simulink model "PickLead_Test"  (Simulink 7.8)
settings: Solver=ode45  StartTime=0.0  StopTime=50  RelTol=1e-3
libraries: simulink x1
settings Model: Creator=jmapatel  LastModifiedBy=cjzhang
settings OptimizationCC: InitFltsAndDblsToZero=on
settings DebuggingCC: SaveWithParameterizedLinksMsg=none  FcnCallInpInsideContextMsg=Use local settings  StrictBusMsg=Warning
settings GRTTargetCC: TargetFcnLib=ansi_tfl_tmw.mat

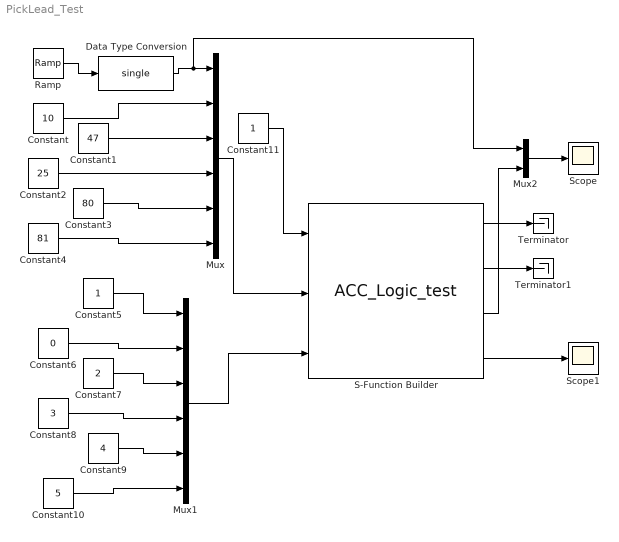
== system PickLead_Test ==
  Constant : Constant  Value=10  OutDataTypeStr=single
  Constant1 : Constant  Value=47  OutDataTypeStr=single
  Constant10 : Constant  Value=5  OutDataTypeStr=single
  Constant11 : Constant  OutDataTypeStr=boolean
  Constant2 : Constant  Value=25  OutDataTypeStr=single
  Constant3 : Constant  Value=80  OutDataTypeStr=single
  Constant4 : Constant  Value=81  OutDataTypeStr=single
  Constant5 : Constant  OutDataTypeStr=single
  Constant6 : Constant  Value=0  OutDataTypeStr=single
  Constant7 : Constant  Value=2  OutDataTypeStr=single
  Constant8 : Constant  Value=3  OutDataTypeStr=single
  Constant9 : Constant  Value=4  OutDataTypeStr=single
  Data Type Conversion : DataTypeConversion  OutDataTypeStr=single
  Mux : Mux  Inputs=6
  Mux1 : Mux  Inputs=6
  Mux2 : Mux  Inputs=2
  Ramp : simulink/Sources/Ramp  slope=2  start=0  X0=0
  S-Function Builder : S-Function  InitFcn=try, set_param(gcb,'FunctionName','ACC_Logic_test'), end  FunctionName=ACC_Logic_test  Parameters=1  SFunctionModules=ACC_Logic_test_wrapper  WizardData=DataTag0  EnableBusSupport=off
      mask init:
      | val = [[.9  0.75 0.75 1 1 .9 .9 1]',[1 1 0.75 0.75 .9 .9 1 .9]'];try , sys = get_param(gcb,'SfunBuilderFcnName');if isempty(sys), sys = get_param(gcb,'FunctionName'); end,catch, sys = get_param(gcb,'FunctionName'); end
      settings: CopyFcn=set_param(gcbh,'LinkStatus','none')  PreSaveFcn=try, set_param(gcb,'FunctionName','ACC_Logic_test'), end  OpenFcn=sfunctionwizard(gcbh)
      mask Display: plot(val(:,1),val(:,2)),disp(sys), port_label('input',1,'en_man'), port_label('input',2,'s'), port_label('input',3,'u'), port_label('output',1,'en_vel'), port_label('output',2,'en_pos'), port_label('output',3,'lead_s'), port_label('output',4,'lead_us')
  Scope : Scope
  Scope1 : Scope
  Terminator : Terminator
  Terminator1 : Terminator
  wires:
  Mux2/1 -> Scope/1
  Constant/1 -> Mux/2
  Constant1/1 -> Mux/3
  Constant2/1 -> Mux/4
  Constant3/1 -> Mux/5
  Constant4/1 -> Mux/6
  Constant5/1 -> Mux1/1
  Constant6/1 -> Mux1/2
  Constant7/1 -> Mux1/3
  Constant8/1 -> Mux1/4
  Constant9/1 -> Mux1/5
  Constant10/1 -> Mux1/6
  Ramp/1 -> Data Type Conversion/1
  Data Type Conversion/1 -> Mux/1, Mux2/1
  Mux/1 -> S-Function Builder/2
  Mux1/1 -> S-Function Builder/3
  Constant11/1 -> S-Function Builder/1
  S-Function Builder/3 -> Mux2/2
  S-Function Builder/4 -> Scope1/1
  S-Function Builder/1 -> Terminator/1
  S-Function Builder/2 -> Terminator1/1
